simulink model "mce"  (Simulink 6.5)
settings: Solver=ode45  StartTime=0.0  StopTime=10.0  RelTol=1e-3
libraries: cdsFilt x334, cdsMatrix x9, cdsSwitch x7, cdsWD x7, cdsMuxMatrix x5, dac x3, cdsEpicsOut x2, cdsParameters x1
(part 1 of 18)
settings Model: Creator=controls  LastModifiedBy=controls  ExtModeAutoUpdateStatusClock=off

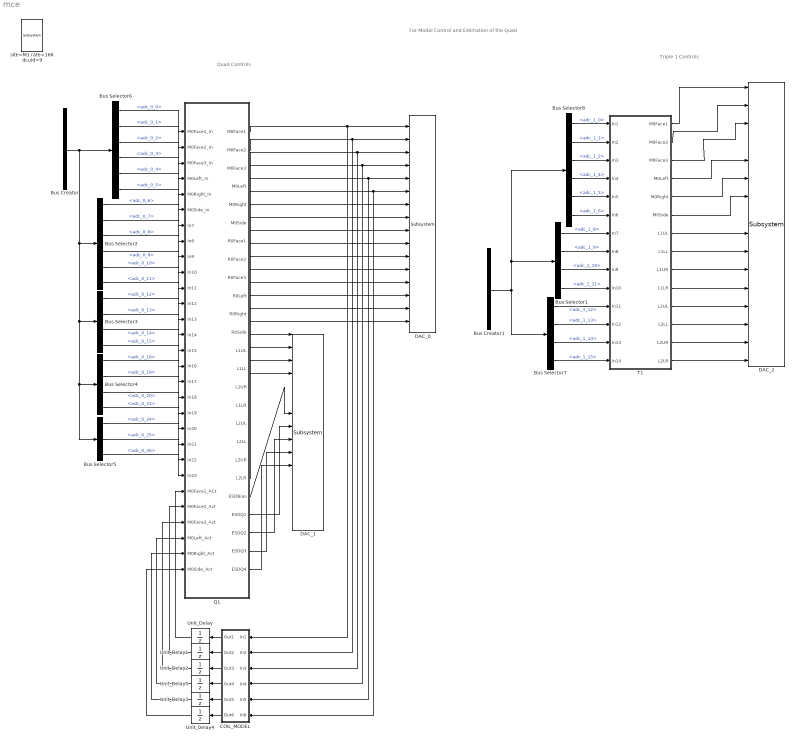
== system mce ==
  note: Triple 1 Controls
  note: Quad Controls
  note: For Modal Control and Estimation of the Quad
  Bus Creator : BusCreator  Tag=adc_0  Description=ADC0  Inputs='adc_0_0','adc_0_1','adc_0_2','adc_0_3','adc_0_4','adc_0_5','adc_0_6','adc_0_7','adc_0_8','adc_0_9','adc_0_10','adc_0_11','adc_0_12','adc_0_13','adc_0_14','adc_0_15','adc_0_16','adc_0_17','adc_0_18','adc_0_19','adc_0_20','adc_0_21','adc_0_22','adc_0_23','adc_0_24','adc_0_25','adc_0_26','adc_0_27','adc_0_28','adc_0_29','adc_0_30','adc_0_31'
      settings: AttributesFormatString=%<Tag>
  Bus Creator1 : BusCreator  Tag=adc_1  Description=|  Inputs='adc_1_0','adc_1_1','adc_1_2','adc_1_3','adc_1_4','adc_1_5','adc_1_6','adc_1_7','adc_1_8','adc_1_9','adc_1_10','adc_1_11','adc_1_12','adc_1_13','adc_1_14','adc_1_15','adc_1_16','adc_1_17','adc_1_18','adc_1_19','adc_1_20','adc_1_21','adc_1_22','adc_1_23','adc_1_24','adc_1_25','adc_1_26','adc_1_27','adc_1_28','adc_1_29','adc_1_30','adc_1_31'
      | PCI66-16AI64SSA
      | 40Vp-p, 16-bit, 610uV/count
      settings: AttributesFormatString=%<Description>\n%<Tag>
  Bus Selector1 : BusSelector  OutputSignals=adc_1_8,adc_1_9,adc_1_10,adc_1_11
  Bus Selector2 : BusSelector  OutputSignals=adc_0_6,adc_0_7,adc_0_8,adc_0_9,adc_0_10,adc_0_11
  Bus Selector3 : BusSelector  OutputSignals=adc_0_12,adc_0_13,adc_0_14,adc_0_15
  Bus Selector4 : BusSelector  OutputSignals=adc_0_18,adc_0_19,adc_0_20,adc_0_21
  Bus Selector5 : BusSelector  OutputSignals=adc_0_24,adc_0_25,adc_0_26
  Bus Selector6 : BusSelector  Description=ADC Selector  OutputSignals=adc_0_0,adc_0_1,adc_0_2,adc_0_3,adc_0_4,adc_0_5
      settings: AttributesFormatString=%<Description>
  Bus Selector7 : BusSelector  OutputSignals=adc_1_12,adc_1_13,adc_1_14,adc_1_15
  Bus Selector8 : BusSelector  OutputSignals=adc_1_0,adc_1_1,adc_1_2,adc_1_4,adc_1_5,adc_1_6
  COIL_MODEL : Subsystem  Orientation=left
  DAC_0 : dac/Subsystem  Description=DAC  SystemSampleTime=-1
      settings: AttributesFormatString=%<Description>
  DAC_1 : dac/Subsystem  Description=|  SystemSampleTime=-1
      | PCI66-16AO16
      | 20Vp-p, 16-bit, 305uV/count
      settings: AttributesFormatString=%<Description>
  DAC_2 : dac/Subsystem  Tag=dac_2  Description=|  SystemSampleTime=-1
      | PCI66-16AO16
      | 20Vp-p, 16-bit, 305uV/count
      settings: AttributesFormatString=%<Description>
  Q1 : Subsystem  Description=Quad Suspension
      settings: AttributesFormatString=%<Description>
  T1 : Subsystem  Description=Triple Suspension
      settings: AttributesFormatString=%<Description>
  Unit_Delay{,1..5} (6 alike) : UnitDelay  Orientation=left
  site=M1 rate=16K dcuid=9 : cdsParameters/Subsystem  Tag=cdsParameters  Description=|  SystemSampleTime=-1
      | Purpose:                                                                                                                                                                                                                                
      | Provide system parameters to the FE code generator to properly configure the generated EPICS names, rep rate of the FE controller, and the Data Acquisition node ID for proper storage of data from this FE controller.                 
      |                                                                                                                                                                                                                                         
      | Useage:                                                                                                                                                                                                                                 
      | The part NAME field is used to identify the FE parameters. It must be of the form:                                                                                                                                                      
      | site=                                                                                                                                                                                                                                   
      | rate=                                                                                                                                                                                                                                   
      | dcuid=                                                                                                                                                                                                                                  
      |                                                                                                                                                                                                                                         
      | Where:                                                                                                                                                                                                                                  
      | site= argument may be H1, H2, L1, M1, G1, either as a single argument or multiple, for example site=H1,H2. These are the only names allowed. These will become the first two characters of all EPICS and signal names (for example G1:).
      |                                                                                                                                                                                                                                         
      | rate= may be 2K, 16K, 32K, or 64K                                                                                                                                                                                                       
      |                                                                                                                                                                                                                                         
      | dcuid= is site specific ie it must be unique at each site.
      settings: AttributesFormatString=%<Tag>
  wires:
  Bus Creator/1 -> Bus Selector6/1, Bus Selector2/1, Bus Selector3/1, Bus Selector4/1, Bus Selector5/1
  T1/1(M0Face1) -> DAC_2/1
  T1/2(M0Face2) -> DAC_2/2
  T1/3(M0Face3) -> DAC_2/3
  T1/4(M0Left) -> DAC_2/5
  T1/5(M0Right) -> DAC_2/6
  T1/6(M0Side) -> DAC_2/7
  Bus Selector8/1 -> T1/1(In1)  "<adc_1_0>"
  Bus Selector8/2 -> T1/2(In2)  "<adc_1_1>"
  Bus Selector8/3 -> T1/3(In3)  "<adc_1_2>"
  Bus Selector8/4 -> T1/4(In4)  "<adc_1_4>"
  Bus Selector8/5 -> T1/5(In5)  "<adc_1_5>"
  Bus Selector8/6 -> T1/6(In6)  "<adc_1_6>"
  Bus Selector1/1 -> T1/7(In7)  "<adc_1_8>"
  Bus Selector1/2 -> T1/8(In8)  "<adc_1_9>"
  Bus Selector1/3 -> T1/9(In9)  "<adc_1_10>"
  Bus Selector1/4 -> T1/10(In10)  "<adc_1_11>"
  Bus Selector7/1 -> T1/11(In11)  "<adc_1_12>"
  Bus Selector7/2 -> T1/12(In12)  "<adc_1_13>"
  Bus Selector7/3 -> T1/13(In13)  "<adc_1_14>"
  Bus Selector7/4 -> T1/14(In14)  "<adc_1_15>"
  Bus Creator1/1 -> Bus Selector7/1, Bus Selector1/1, Bus Selector8/1
  T1/14(L2LR) -> DAC_2/16
  T1/13(L2UR) -> DAC_2/15
  T1/12(L2LL) -> DAC_2/14
  T1/11(L2UL) -> DAC_2/13
  T1/10(L1LR) -> DAC_2/12
  T1/9(L1UR) -> DAC_2/11
  T1/8(L1LL) -> DAC_2/10
  T1/7(L1UL) -> DAC_2/9
  Bus Selector2/1 -> Q1/7(In7)  "<adc_0_6>"
  Bus Selector6/1 -> Q1/1(M0Face1_In)  "<adc_0_0>"
  Bus Selector6/2 -> Q1/2(M0Face2_In)  "<adc_0_1>"
  Bus Selector6/3 -> Q1/3(M0Face3_In)  "<adc_0_2>"
  Bus Selector6/4 -> Q1/4(M0Left_In)  "<adc_0_3>"
  Bus Selector6/5 -> Q1/5(M0Right_In)  "<adc_0_4>"
  Bus Selector6/6 -> Q1/6(M0Side_In)  "<adc_0_5>"
  Bus Selector3/1 -> Q1/13(In13)  "<adc_0_12>"
  Bus Selector3/2 -> Q1/14(In14)  "<adc_0_13>"
  Bus Selector3/3 -> Q1/15(In15)  "<adc_0_14>"
  Bus Selector3/4 -> Q1/16(In16)  "<adc_0_15>"
  Bus Selector4/1 -> Q1/17(In17)  "<adc_0_18>"
  Bus Selector4/2 -> Q1/18(In18)  "<adc_0_19>"
  Bus Selector4/3 -> Q1/19(In19)  "<adc_0_20>"
  Bus Selector4/4 -> Q1/20(In20)  "<adc_0_21>"
  Bus Selector5/1 -> Q1/21(In21)  "<adc_0_24>"
  Bus Selector5/2 -> Q1/22(In22)  "<adc_0_25>"
  Bus Selector5/3 -> Q1/23(In23)  "<adc_0_26>"
  Q1/1(M0Face1) -> DAC_0/1, COIL_MODEL/1(In1)
  Q1/2(M0Face2) -> DAC_0/2, COIL_MODEL/2(In2)
  Q1/3(M0Face3) -> DAC_0/3, COIL_MODEL/3(In3)
  Q1/4(M0Left) -> DAC_0/4, COIL_MODEL/4(In4)
  Q1/5(M0Right) -> DAC_0/5, COIL_MODEL/5(In5)
  Q1/6(M0Side) -> DAC_0/6, COIL_MODEL/6(In6)
  Q1/7(R0Face1) -> DAC_0/7
  Q1/8(R0Face2) -> DAC_0/8
  Q1/9(R0Face3) -> DAC_0/9
  Q1/10(R0Left) -> DAC_0/10
  Q1/11(R0Right) -> DAC_0/11
  Q1/12(R0Side) -> DAC_0/12
  Q1/13(L1UL) -> DAC_0/13
  Q1/14(L1LL) -> DAC_0/14
  Q1/15(L1UR) -> DAC_0/15
  Q1/16(L1LR) -> DAC_0/16
  Q1/17(L2UL) -> DAC_1/1
  Q1/18(L2LL) -> DAC_1/2
  Q1/19(L2UR) -> DAC_1/3
  Q1/20(L2LR) -> DAC_1/4
  Q1/21(ESDBias) -> DAC_1/7
  Q1/22(ESDQ1) -> DAC_1/8
  Q1/23(ESDQ2) -> DAC_1/9
  Q1/24(ESDQ3) -> DAC_1/10
  Q1/25(ESDQ4) -> DAC_1/11
  Bus Selector2/2 -> Q1/8(In8)  "<adc_0_7>"
  Bus Selector2/3 -> Q1/9(In9)  "<adc_0_8>"
  Bus Selector2/4 -> Q1/10(In10)  "<adc_0_9>"
  Bus Selector2/5 -> Q1/11(In11)  "<adc_0_10>"
  Bus Selector2/6 -> Q1/12(In12)  "<adc_0_11>"
  COIL_MODEL/1(Out1) -> Unit_Delay/1
  Unit_Delay/1 -> Q1/24(M0Face1_ACt)
  COIL_MODEL/2(Out2) -> Unit_Delay1/1
  Unit_Delay1/1 -> Q1/25(M0Face2_Act)
  COIL_MODEL/3(Out3) -> Unit_Delay2/1
  Unit_Delay2/1 -> Q1/26(M0Face3_Act)
  COIL_MODEL/4(Out4) -> Unit_Delay5/1
  Unit_Delay5/1 -> Q1/27(M0Left_Act)
  COIL_MODEL/5(Out5) -> Unit_Delay3/1
  Unit_Delay3/1 -> Q1/28(M0Right_Act)
  COIL_MODEL/6(Out6) -> Unit_Delay4/1
  Unit_Delay4/1 -> Q1/29(M0Side_Act)

== system mce/COIL_MODEL ==
  In1 : Inport  Orientation=left
  In2 : Inport  Orientation=left  Port=2
  In3 : Inport  Orientation=left  Port=3
  In4 : Inport  Orientation=left  Port=4
  In5 : Inport  Orientation=left  Port=5
  In6 : Inport  Orientation=left  Port=6
  F1_COIL : cdsFilt/Subsystem  Tag=cdsFilt  Description=|  Orientation=left  SystemSampleTime=-1
      | Purpose:                                                                                                                                                                                                                                  
      | Standard CDS IIR filter module.                                                                                                                                                                                                           
      |                                                                                                                                                                                                                                           
      | Operation:                                                                                                                                                                                                                                
      | Consists of 10 second order section IIR filters, plus a ramped gain stage. In FE code, also provides pre-defined test points and excitation channel inputs. The filter coefficients are defined in the LIGO system using the 'foton' tool.
      |                                                                                                                                                                                                                                           
      | Usage:                                                                                                                                                                                                                                    
      | Name the part with the desired filter module name.
      settings: AttributesFormatString=%<Tag>
  F2_COIL : cdsFilt/Subsystem  Tag=cdsFilt  Description=|  Orientation=left  SystemSampleTime=-1
      | Purpose:                                                                                                                                                                                                                                  
      | Standard CDS IIR filter module.                                                                                                                                                                                                           
      |                                                                                                                                                                                                                                           
      | Operation:                                                                                                                                                                                                                                
      | Consists of 10 second order section IIR filters, plus a ramped gain stage. In FE code, also provides pre-defined test points and excitation channel inputs. The filter coefficients are defined in the LIGO system using the 'foton' tool.
      |                                                                                                                                                                                                                                           
      | Usage:                                                                                                                                                                                                                                    
      | Name the part with the desired filter module name.
      settings: AttributesFormatString=%<Tag>
  F3_COIL : cdsFilt/Subsystem  Tag=cdsFilt  Description=|  Orientation=left  SystemSampleTime=-1
      | Purpose:                                                                                                                                                                                                                                  
      | Standard CDS IIR filter module.                                                                                                                                                                                                           
      |                                                                                                                                                                                                                                           
      | Operation:                                                                                                                                                                                                                                
      | Consists of 10 second order section IIR filters, plus a ramped gain stage. In FE code, also provides pre-defined test points and excitation channel inputs. The filter coefficients are defined in the LIGO system using the 'foton' tool.
      |                                                                                                                                                                                                                                           
      | Usage:                                                                                                                                                                                                                                    
      | Name the part with the desired filter module name.
      settings: AttributesFormatString=%<Tag>
  L_COIL : cdsFilt/Subsystem  Tag=cdsFilt  Description=|  Orientation=left  SystemSampleTime=-1
      | Purpose:                                                                                                                                                                                                                                  
      | Standard CDS IIR filter module.                                                                                                                                                                                                           
      |                                                                                                                                                                                                                                           
      | Operation:                                                                                                                                                                                                                                
      | Consists of 10 second order section IIR filters, plus a ramped gain stage. In FE code, also provides pre-defined test points and excitation channel inputs. The filter coefficients are defined in the LIGO system using the 'foton' tool.
      |                                                                                                                                                                                                                                           
      | Usage:                                                                                                                                                                                                                                    
      | Name the part with the desired filter module name.
      settings: AttributesFormatString=%<Tag>
  R_COIL : cdsFilt/Subsystem  Tag=cdsFilt  Description=|  Orientation=left  SystemSampleTime=-1
      | Purpose:                                                                                                                                                                                                                                  
      | Standard CDS IIR filter module.                                                                                                                                                                                                           
      |                                                                                                                                                                                                                                           
      | Operation:                                                                                                                                                                                                                                
      | Consists of 10 second order section IIR filters, plus a ramped gain stage. In FE code, also provides pre-defined test points and excitation channel inputs. The filter coefficients are defined in the LIGO system using the 'foton' tool.
      |                                                                                                                                                                                                                                           
      | Usage:                                                                                                                                                                                                                                    
      | Name the part with the desired filter module name.
      settings: AttributesFormatString=%<Tag>
  S_COIL : cdsFilt/Subsystem  Tag=cdsFilt  Description=|  Orientation=left  SystemSampleTime=-1
      | Purpose:                                                                                                                                                                                                                                  
      | Standard CDS IIR filter module.                                                                                                                                                                                                           
      |                                                                                                                                                                                                                                           
      | Operation:                                                                                                                                                                                                                                
      | Consists of 10 second order section IIR filters, plus a ramped gain stage. In FE code, also provides pre-defined test points and excitation channel inputs. The filter coefficients are defined in the LIGO system using the 'foton' tool.
      |                                                                                                                                                                                                                                           
      | Usage:                                                                                                                                                                                                                                    
      | Name the part with the desired filter module name.
      settings: AttributesFormatString=%<Tag>
  Out1 : Outport  Orientation=left
  Out2 : Outport  Orientation=left  Port=2
  Out3 : Outport  Orientation=left  Port=3
  Out4 : Outport  Orientation=left  Port=4
  Out5 : Outport  Orientation=left  Port=5
  Out6 : Outport  Orientation=left  Port=6
  wires:
  In1/1 -> F1_COIL/1
  In2/1 -> F2_COIL/1
  In3/1 -> F3_COIL/1
  In4/1 -> L_COIL/1
  In5/1 -> R_COIL/1
  In6/1 -> S_COIL/1
  F1_COIL/1 -> Out1/1
  F2_COIL/1 -> Out2/1
  F3_COIL/1 -> Out3/1
  L_COIL/1 -> Out4/1
  R_COIL/1 -> Out5/1
  S_COIL/1 -> Out6/1

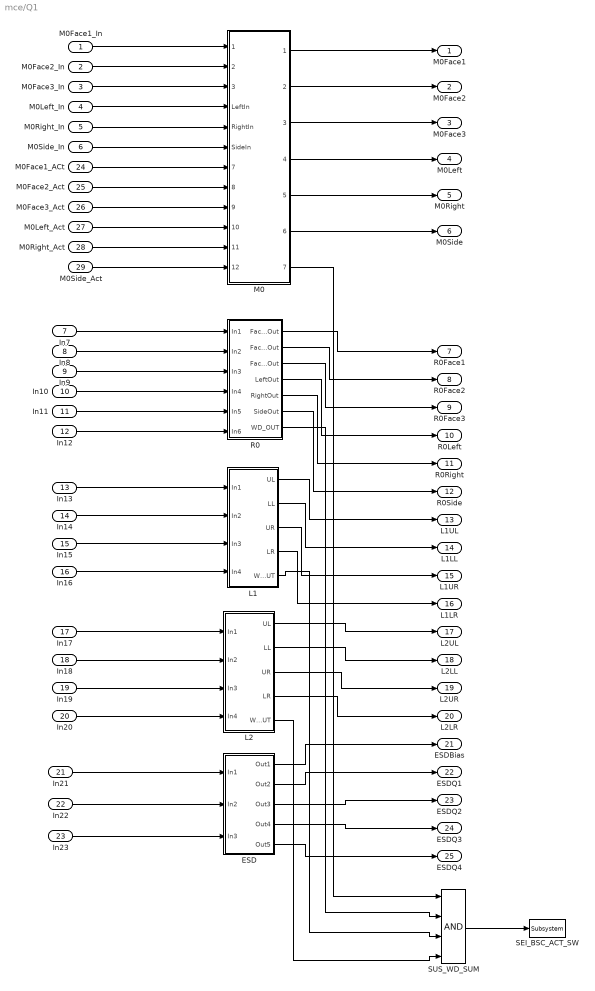
== system mce/Q1 ==
  M0Face1_In : Inport
  M0Face2_In : Inport  Port=2
  M0Face3_In : Inport  Port=3
  M0Left_In : Inport  Port=4
  M0Right_In : Inport  Port=5
  M0Side_In : Inport  Port=6
  In7 : Inport  Port=7
  In8 : Inport  Port=8
  In9 : Inport  Port=9
  In10 : Inport  Port=10
  In11 : Inport  Port=11
  In12 : Inport  Port=12
  In13 : Inport  Port=13
  In14 : Inport  Port=14
  In15 : Inport  Port=15
  In16 : Inport  Port=16
  In17 : Inport  Port=17
  In18 : Inport  Port=18
  In19 : Inport  Port=19
  In20 : Inport  Port=20
  In21 : Inport  Port=21
  In22 : Inport  Port=22
  In23 : Inport  Port=23
  M0Face1_ACt : Inport  Port=24
  M0Face2_Act : Inport  Port=25
  M0Face3_Act : Inport  Port=26
  M0Left_Act : Inport  Port=27
  M0Right_Act : Inport  Port=28
  M0Side_Act : Inport  Port=29
  ESD : Subsystem
  L1 : Subsystem
  L2 : Subsystem
  M0 : Subsystem
  R0 : Subsystem
  SEI_BSC_ACT_SW : cdsEpicsOut/Subsystem  Tag=cdsEpicsOutput  Description=|  SystemSampleTime=-1
      | Purpose:                                          
      | Output a FE signal to an EPICS channel.           
      |                                                   
      | Operation:                                        
      | Takes input value and passes it to EPICS record.  
      |                                                   
      | Usage:                                            
      | Name the part with the desired EPICS rrecord name.
      settings: AttributesFormatString=%<Tag>
  SUS_WD_SUM : Logic  Inputs=4  AllPortsSameDT=off  OutDataTypeMode=Boolean
  M0Face1 : Outport
  M0Face2 : Outport  Port=2
  M0Face3 : Outport  Port=3
  M0Left : Outport  Port=4
  M0Right : Outport  Port=5
  M0Side : Outport  Port=6
  R0Face1 : Outport  Port=7
  R0Face2 : Outport  Port=8
  R0Face3 : Outport  Port=9
  R0Left : Outport  Port=10
  R0Right : Outport  Port=11
  R0Side : Outport  Port=12
  L1UL : Outport  Port=13
  L1LL : Outport  Port=14
  L1UR : Outport  Port=15
  L1LR : Outport  Port=16
  L2UL : Outport  Port=17
  L2LL : Outport  Port=18
  L2UR : Outport  Port=19
  L2LR : Outport  Port=20
  ESDBias : Outport  Port=21
  ESDQ1 : Outport  Port=22
  ESDQ2 : Outport  Port=23
  ESDQ3 : Outport  Port=24
  ESDQ4 : Outport  Port=25
  wires:
  SUS_WD_SUM/1 -> SEI_BSC_ACT_SW/1
  R0/7(WD_OUT) -> SUS_WD_SUM/2
  L1/5(WD_OUT) -> SUS_WD_SUM/3
  L2/5(WD_OUT) -> SUS_WD_SUM/4
  In7/1 -> R0/1(In1)
  In8/1 -> R0/2(In2)
  In9/1 -> R0/3(In3)
  In10/1 -> R0/4(In4)
  In11/1 -> R0/5(In5)
  In12/1 -> R0/6(In6)
  In13/1 -> L1/1(In1)
  In14/1 -> L1/2(In2)
  In15/1 -> L1/3(In3)
  In16/1 -> L1/4(In4)
  In17/1 -> L2/1(In1)
  In18/1 -> L2/2(In2)
  In19/1 -> L2/3(In3)
  In20/1 -> L2/4(In4)
  In21/1 -> ESD/1(In1)
  In22/1 -> ESD/2(In2)
  In23/1 -> ESD/3(In3)
  R0/1(Face1Out) -> R0Face1/1
  R0/2(Face2Out) -> R0Face2/1
  R0/3(Face3Out) -> R0Face3/1
  R0/4(LeftOut) -> R0Left/1
  R0/6(SideOut) -> R0Side/1
  L1/1(UL) -> L1UL/1
  L1/2(LL) -> L1LL/1
  L1/3(UR) -> L1UR/1
  L1/4(LR) -> L1LR/1
  ESD/1(Out1) -> ESDBias/1
  ESD/2(Out2) -> ESDQ1/1
  ESD/3(Out3) -> ESDQ2/1
  ESD/4(Out4) -> ESDQ3/1
  ESD/5(Out5) -> ESDQ4/1
  R0/5(RightOut) -> R0Right/1
  L2/1(UL) -> L2UL/1
  L2/2(LL) -> L2LL/1
  L2/3(UR) -> L2UR/1
  L2/4(LR) -> L2LR/1
  M0/1(Face1Out) -> M0Face1/1
  M0/2(Face2Out) -> M0Face2/1
  M0/3(Face3Out) -> M0Face3/1
  M0/4(LeftOut) -> M0Left/1
  M0/5(RightOut) -> M0Right/1
  M0/6(SideOut) -> M0Side/1
  M0/7(WD_Out) -> SUS_WD_SUM/1
  M0Face3_In/1 -> M0/3(Face3In)
  M0Left_In/1 -> M0/4(LeftIn)
  M0Right_In/1 -> M0/5(RightIn)
  M0Side_In/1 -> M0/6(SideIn)
  M0Face1_ACt/1 -> M0/7(Face1_Act)
  M0Face2_Act/1 -> M0/8(Face2_ACT)
  M0Face3_Act/1 -> M0/9(Face3_Act)
  M0Left_Act/1 -> M0/10(Left_Act)
  M0Right_Act/1 -> M0/11(Right_Act)
  M0Side_Act/1 -> M0/12(Side_Act)
  M0Face2_In/1 -> M0/2(Face2In)
  M0Face1_In/1 -> M0/1(Face1In)

== system mce/T1 ==
  In1 : Inport
  In2 : Inport  Port=2
  In3 : Inport  Port=3
  In4 : Inport  Port=4
  In5 : Inport  Port=5
  In6 : Inport  Port=6
  In7 : Inport  Port=7
  In8 : Inport  Port=8
  In9 : Inport  Port=9
  In10 : Inport  Port=10
  In11 : Inport  Port=11
  In12 : Inport  Port=12
  In13 : Inport  Port=13
  In14 : Inport  Port=14
  L1 : Subsystem
  L2 : Subsystem
  M0 : Subsystem
  SEI_HAMY_ACT_SW : cdsEpicsOut/Subsystem  Tag=cdsEpicsOutput  Description=|  SystemSampleTime=-1
      | Purpose:                                          
      | Output a FE signal to an EPICS channel.           
      |                                                   
      | Operation:                                        
      | Takes input value and passes it to EPICS record.  
      |                                                   
      | Usage:                                            
      | Name the part with the desired EPICS rrecord name.
      settings: AttributesFormatString=%<Tag>
  SUS_WD_SUM : Logic  Inputs=3  AllPortsSameDT=off  OutDataTypeMode=Boolean
  M0Face1 : Outport
  M0Face2 : Outport  Port=2
  M0Face3 : Outport  Port=3
  M0Left : Outport  Port=4
  M0Right : Outport  Port=5
  M0Side : Outport  Port=6
  L1UL : Outport  Port=7
  L1LL : Outport  Port=8
  L1UR : Outport  Port=9
  L1LR : Outport  Port=10
  L2UL : Outport  Port=11
  L2LL : Outport  Port=12
  L2UR : Outport  Port=13
  L2LR : Outport  Port=14
  wires:
  M0/1(Face1Out) -> M0Face1/1
  M0/2(Face2Out) -> M0Face2/1
  M0/3(Face3Out) -> M0Face3/1
  M0/4(LeftOut) -> M0Left/1
  M0/5(RightOut) -> M0Right/1
  M0/6(SideOut) -> M0Side/1
  SUS_WD_SUM/1 -> SEI_HAMY_ACT_SW/1
  M0/7(WD_OUT) -> SUS_WD_SUM/1
  L1/5(WD_OUT) -> SUS_WD_SUM/2
  L2/5(WD_OUT) -> SUS_WD_SUM/3
  In1/1 -> M0/1(In1)
  In2/1 -> M0/2(In2)
  In3/1 -> M0/3(In3)
  In4/1 -> M0/4(In4)
  In5/1 -> M0/5(In5)
  In6/1 -> M0/6(In6)
  In7/1 -> L1/1(In1)
  In8/1 -> L1/2(In2)
  In9/1 -> L1/3(In3)
  In10/1 -> L1/4(In4)
  In11/1 -> L2/1(In1)
  In12/1 -> L2/2(In2)
  In13/1 -> L2/3(In3)
  In14/1 -> L2/4(In4)
  L1/1(UL) -> L1UL/1
  L1/2(LL) -> L1LL/1
  L1/3(UR) -> L1UR/1
  L1/4(LR) -> L1LR/1
  L2/1(UL) -> L2UL/1
  L2/2(LL) -> L2LL/1
  L2/3(UR) -> L2UR/1
  L2/4(LR) -> L2LR/1

== system mce/Q1/ESD ==
  In1 : Inport
  In2 : Inport  Port=2
  In3 : Inport  Port=3
  ASCP : cdsFilt/Subsystem  Tag=cdsFilt  Description=|  SystemSampleTime=-1
      | Purpose:                                                                                                                                                                                                                                  
      | Standard CDS IIR filter module.                                                                                                                                                                                                           
      |                                                                                                                                                                                                                                           
      | Operation:                                                                                                                                                                                                                                
      | Consists of 10 second order section IIR filters, plus a ramped gain stage. In FE code, also provides pre-defined test points and excitation channel inputs. The filter coefficients are defined in the LIGO system using the 'foton' tool.
      |                                                                                                                                                                                                                                           
      | Usage:                                                                                                                                                                                                                                    
      | Name the part with the desired filter module name.
      settings: AttributesFormatString=%<Tag>
  ASCY : cdsFilt/Subsystem  Tag=cdsFilt  Description=|  SystemSampleTime=-1
      | Purpose:                                                                                                                                                                                                                                  
      | Standard CDS IIR filter module.                                                                                                                                                                                                           
      |                                                                                                                                                                                                                                           
      | Operation:                                                                                                                                                                                                                                
      | Consists of 10 second order section IIR filters, plus a ramped gain stage. In FE code, also provides pre-defined test points and excitation channel inputs. The filter coefficients are defined in the LIGO system using the 'foton' tool.
      |                                                                                                                                                                                                                                           
      | Usage:                                                                                                                                                                                                                                    
      | Name the part with the desired filter module name.
      settings: AttributesFormatString=%<Tag>
  BIAS : cdsFilt/Subsystem  Tag=cdsFilt  Description=|  SystemSampleTime=-1
      | Purpose:                                                                                                                                                                                                                                  
      | Standard CDS IIR filter module.                                                                                                                                                                                                           
      |                                                                                                                                                                                                                                           
      | Operation:                                                                                                                                                                                                                                
      | Consists of 10 second order section IIR filters, plus a ramped gain stage. In FE code, also provides pre-defined test points and excitation channel inputs. The filter coefficients are defined in the LIGO system using the 'foton' tool.
      |                                                                                                                                                                                                                                           
      | Usage:                                                                                                                                                                                                                                    
      | Name the part with the desired filter module name.
      settings: AttributesFormatString=%<Tag>
  INMTRX : cdsMatrix/Subsystem  Tag=Matrix  Description=|  SystemSampleTime=-1
      | Purpose:                                                                 
      | Provide a matrix multiplication function for up to 8 input and 8 outputs.
      settings: AttributesFormatString=%<Tag>
  LSC : cdsFilt/Subsystem  Tag=cdsFilt  Description=|  SystemSampleTime=-1
      | Purpose:                                                                                                                                                                                                                                  
      | Standard CDS IIR filter module.                                                                                                                                                                                                           
      |                                                                                                                                                                                                                                           
      | Operation:                                                                                                                                                                                                                                
      | Consists of 10 second order section IIR filters, plus a ramped gain stage. In FE code, also provides pre-defined test points and excitation channel inputs. The filter coefficients are defined in the LIGO system using the 'foton' tool.
      |                                                                                                                                                                                                                                           
      | Usage:                                                                                                                                                                                                                                    
      | Name the part with the desired filter module name.
      settings: AttributesFormatString=%<Tag>
  Q1 : cdsFilt/Subsystem  Tag=cdsFilt  Description=|  SystemSampleTime=-1
      | Purpose:                                                                                                                                                                                                                                  
      | Standard CDS IIR filter module.                                                                                                                                                                                                           
      |                                                                                                                                                                                                                                           
      | Operation:                                                                                                                                                                                                                                
      | Consists of 10 second order section IIR filters, plus a ramped gain stage. In FE code, also provides pre-defined test points and excitation channel inputs. The filter coefficients are defined in the LIGO system using the 'foton' tool.
      |                                                                                                                                                                                                                                           
      | Usage:                                                                                                                                                                                                                                    
      | Name the part with the desired filter module name.
      settings: AttributesFormatString=%<Tag>
  Q2 : cdsFilt/Subsystem  Tag=cdsFilt  Description=|  SystemSampleTime=-1
      | Purpose:                                                                                                                                                                                                                                  
      | Standard CDS IIR filter module.                                                                                                                                                                                                           
      |                                                                                                                                                                                                                                           
      | Operation:                                                                                                                                                                                                                                
      | Consists of 10 second order section IIR filters, plus a ramped gain stage. In FE code, also provides pre-defined test points and excitation channel inputs. The filter coefficients are defined in the LIGO system using the 'foton' tool.
      |                                                                                                                                                                                                                                           
      | Usage:                                                                                                                                                                                                                                    
      | Name the part with the desired filter module name.
      settings: AttributesFormatString=%<Tag>
  Q3 : cdsFilt/Subsystem  Tag=cdsFilt  Description=|  SystemSampleTime=-1
      | Purpose:                                                                                                                                                                                                                                  
      | Standard CDS IIR filter module.                                                                                                                                                                                                           
      |                                                                                                                                                                                                                                           
      | Operation:                                                                                                                                                                                                                                
      | Consists of 10 second order section IIR filters, plus a ramped gain stage. In FE code, also provides pre-defined test points and excitation channel inputs. The filter coefficients are defined in the LIGO system using the 'foton' tool.
      |                                                                                                                                                                                                                                           
      | Usage:                                                                                                                                                                                                                                    
      | Name the part with the desired filter module name.
      settings: AttributesFormatString=%<Tag>
  Q4 : cdsFilt/Subsystem  Tag=cdsFilt  Description=|  SystemSampleTime=-1
      | Purpose:                                                                                                                                                                                                                                  
      | Standard CDS IIR filter module.                                                                                                                                                                                                           
      |                                                                                                                                                                                                                                           
      | Operation:                                                                                                                                                                                                                                
      | Consists of 10 second order section IIR filters, plus a ramped gain stage. In FE code, also provides pre-defined test points and excitation channel inputs. The filter coefficients are defined in the LIGO system using the 'foton' tool.
      |                                                                                                                                                                                                                                           
      | Usage:                                                                                                                                                                                                                                    
      | Name the part with the desired filter module name.
      settings: AttributesFormatString=%<Tag>
  Out1 : Outport
  Out2 : Outport  Port=2
  Out3 : Outport  Port=3
  Out4 : Outport  Port=4
  Out5 : Outport  Port=5
  wires:
  LSC/1 -> INMTRX/1
  ASCP/1 -> INMTRX/2
  ASCY/1 -> INMTRX/3
  INMTRX/1 -> BIAS/1
  INMTRX/2 -> Q1/1
  INMTRX/3 -> Q2/1
  INMTRX/4 -> Q3/1
  INMTRX/5 -> Q4/1
  BIAS/1 -> Out1/1
  In1/1 -> LSC/1
  Q1/1 -> Out2/1
  In2/1 -> ASCP/1
  Q2/1 -> Out3/1
  In3/1 -> ASCY/1
  Q3/1 -> Out4/1
  Q4/1 -> Out5/1
